simulink model "RCAM_model_Longitudinal"  (R2022b)
settings: Solver=VariableStepAuto  StartTime=0.0  StopTime=10.0  RelTol=1e-3
libraries: cstblocks x1
settings Model: Creator=bendr  LastModifiedBy=bendr

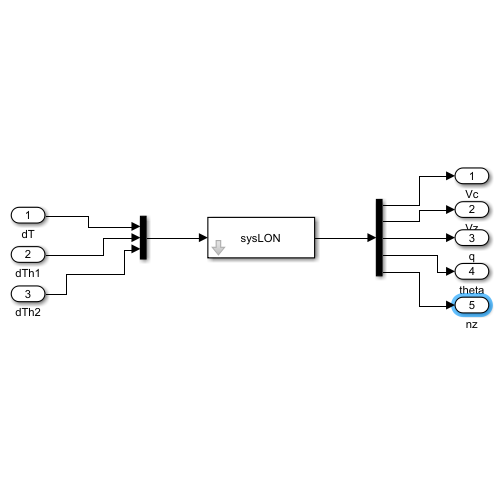
[thumbnail: Simulink's stored preview of the top-level diagram]
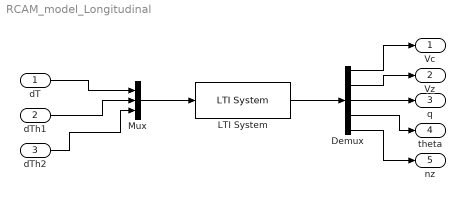
== system RCAM_model_Longitudinal ==
  dT : Inport
  dTh1 : Inport  Port=2
  dTh2 : Inport  Port=3
  Demux : Demux  Outputs=5
  LTI System : cstblocks/LTI System  sys=sysLON  IC=[]
  Mux : Mux  Inputs=3
  Vc : Outport
  Vz : Outport  Port=2
  q : Outport  Port=3
  theta : Outport  Port=4
  nz : Outport  Port=5
  wires:
  dT/1 -> Mux/1
  LTI System/1 -> Demux/1
  Demux/2 -> Vz/1
  Demux/5 -> nz/1
  Demux/1 -> Vc/1
  Mux/1 -> LTI System/1
  Demux/4 -> theta/1
  dTh1/1 -> Mux/2
  Demux/3 -> q/1
  dTh2/1 -> Mux/3
